simulink model "DC_motor_EX2_4"  (R2022a)
settings: Solver=FixedStepDiscrete  StartTime=0.0  StopTime=0.2  FixedStep=Ts  RelTol=1e-3  EnableMultiTasking=on
values from neighbouring files (symbols this model uses):
  Ad = dis_sys.A    [DC_motor.m]
  B_noise1 = [Bd Bw]    [DC_motor.m]
  Bd = dis_sys.B    [DC_motor.m]
  Cd = dis_sys.C    [DC_motor.m]
  D_noise1 = [Dd Dd Dd]    [DC_motor.m]
  N = 10    [DC_motor.m]
  P1 = zeros(size(S))    [DC_motor.m]
  Pr = P    [DC_motor.m]
  Q = 1000*eye(2)    [DC_motor.m]
  QMPC = Q    [DC_motor.m]
  R = R    (= 1)    [DC_motor.m]
  S = P    [DC_motor.m]
  sat_max = Vmax    (= 12)    [DC_motor.m]
  sat_min = Vmin    (= 0)    [DC_motor.m]
  Ts = 1e-3    (= 0.001)    [DC_motor.m]
  Vmax = 12    [DC_motor.m]
  Vmin = 0    [DC_motor.m]
  W = [1 ... (first row only)    [DC_motor.m]
  x0 = [I0 n0]'    [DC_motor.m]
  xmax = [Imax,nmax]'    [DC_motor.m]
  xmin = [Imin,nmin]'    [DC_motor.m]
  xref = [0 0]'    [DC_motor.m]
undefined symbols (not defined in the file or in its folder): MPC_Constrainte, mympc
settings Model: Creator=Mirko  LastModifiedBy=jj
settings SolverCC: AlgebraicLoopSolver=TrustRegion
settings DataIOCC: LimitDataPoints=on  SaveFormat=Array  SignalLoggingSaveFormat=ModelDataLogs  ReturnWorkspaceOutputs=off
settings OptimizationCC: ExpressionDepthLimit=2147483647  LifeSpan=inf
settings DebuggingCC: UnderspecifiedInitializationDetection=Classic  MergeDetectMultiDrivingBlocksExec=none  SolverPrmCheckMsg=warning  FcnCallInpInsideContextMsg=warning  UnconnectedInputMsg=warning  UnconnectedOutputMsg=warning  UnconnectedLineMsg=warning  StateNameClashWarn=warning  SFUnexpectedBacktrackingDiag=warning  SFNoUnconditionalDefaultTransitionDiag=warning  SFExecutionAtInitializationDiag=none  SFMachineParentedDataDiag=warning  ArithmeticOperatorsInVariantConditions=warning
settings HardwareCC: ProdBitPerPointer=32  ProdBitPerSizeT=32  ProdBitPerPtrDiffT=32  ProdLargestAtomicFloat=None  ProdIntDivRoundTo=Undefined  ProdEndianess=Unspecified  ProdWordSize=32  ProdHWDeviceType=32-bit Generic
settings ModelReferenceCC: PropagateSignalLabelsOutOfModel=off
settings SFSimCC: SimUseLocalCustomCode=off  CustomCodeUndefinedFunction=UseInterfaceOnly
settings RTWCC: RTWUseLocalCustomCode=off  DLArmComputeVersion=19.05
settings CodeAppCC: StateflowObjectComments=on
settings GRTTargetCC: TargetLangStandard=C89/C90 (ANSI)
settings ConfigComp: CovMetricSettings=dw  CovSaveCumulativeToWorkspaceVar=on  CovSaveSingleToWorkspaceVar=on  CovExternalEMLEnable=off  CovSFcnEnable=off

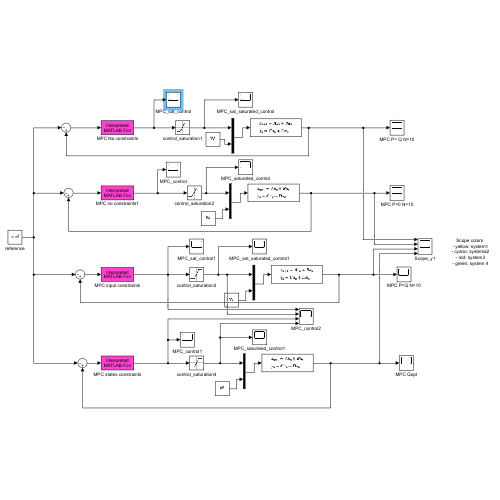
[thumbnail: Simulink's stored preview of the top-level diagram]
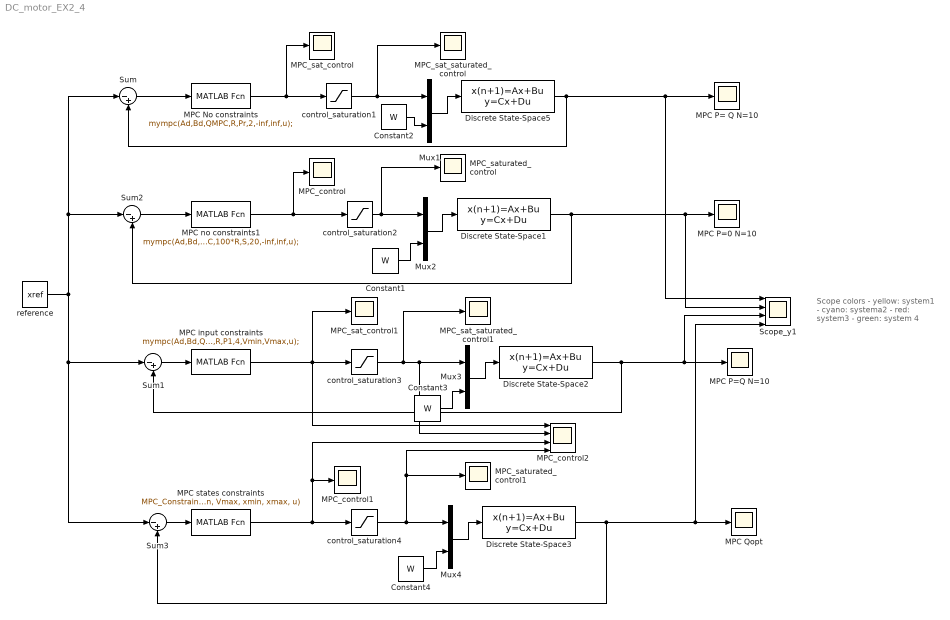
== system DC_motor_EX2_4 ==
  note: Scope colors
      | - yellow: system1
      | - cyano: systema2
      | - red: system3
      | - green: system 4
  Constant{1..4} (4 alike) : Constant  Value=W  SampleTime=Ts
  Discrete State-Space{1..3,5} (4 alike) : DiscreteStateSpace  A=Ad  B=B_noise1  C=Cd  D=D_noise1  InitialCondition=x0  SampleTime=Ts
  MPC No constraints : MATLABFcn  MATLABFcn=mympc(Ad,Bd,QMPC,R,Pr,2,-inf,inf,u);  OutputDimensions=1
  MPC P= Q N=10 : Scope
  MPC P=0 N=10 : Scope
  MPC P=Q N=10 : Scope
  MPC Qopt : Scope
  MPC input constraints : MATLABFcn  MATLABFcn=mympc(Ad,Bd,QMPC,R,P1,4,Vmin,Vmax,u);  OutputDimensions=1
  MPC no constraints1 : MATLABFcn  MATLABFcn=mympc(Ad,Bd,QMPC,100*R,S,20,-inf,inf,u);  OutputDimensions=1
  MPC states constraints : MATLABFcn  MATLABFcn=MPC_Constrainte( Ad,Bd, Q, R, Pr, N, Vmin, Vmax, xmin, xmax, u)  OutputDimensions=1
  MPC_control : Scope
  MPC_control1 : Scope
  MPC_control2 : Scope  NumInputPorts=4
  MPC_sat_control : Scope
  MPC_sat_control1 : Scope
  MPC_sat_saturated_control : Scope
  MPC_sat_saturated_control1 : Scope
  MPC_saturated_control : Scope
  MPC_saturated_control1 : Scope
  Mux{1..4} (4 alike) : Mux  Inputs=2
  Scope_y1 : Scope  NumInputPorts=4
  Sum{,1..3} (4 alike) : Sum  Inputs=|-+
  control_saturation1 : Saturate  UpperLimit=inf  LowerLimit=-inf
  control_saturation2 : Saturate  UpperLimit=inf  LowerLimit=-inf
  control_saturation3 : Saturate  UpperLimit=sat_max  LowerLimit=sat_min
  control_saturation4 : Saturate  UpperLimit=sat_max  LowerLimit=sat_min
  reference : Constant  Value=xref
  wires:
  Sum/1 -> MPC No constraints/1
  MPC No constraints/1 -> control_saturation1/1, MPC_sat_control/1
  Discrete State-Space5/1 -> MPC P= Q N=10/1, Scope_y1/1, Sum/2
  MPC no constraints1/1 -> control_saturation2/1, MPC_control/1
  Discrete State-Space1/1 -> Scope_y1/2, MPC P=0 N=10/1, Sum2/2
  Sum2/1 -> MPC no constraints1/1
  Sum3/1 -> MPC states constraints/1
  control_saturation4/1 -> Mux4/1, MPC_control2/4, MPC_saturated_control1/1
  Discrete State-Space3/1 -> MPC Qopt/1, Scope_y1/4, Sum3/2
  MPC states constraints/1 -> control_saturation4/1, MPC_control2/3, MPC_control1/1
  Discrete State-Space2/1 -> Sum1/2, Scope_y1/3, MPC P=Q N=10/1
  control_saturation3/1 -> Mux3/1, MPC_control2/2, MPC_sat_saturated_control1/1
  MPC input constraints/1 -> MPC_control2/1, control_saturation3/1, MPC_sat_control1/1
  Sum1/1 -> MPC input constraints/1
  reference/1 -> Sum1/1, Sum3/1, Sum/1, Sum2/1
  Mux1/1 -> Discrete State-Space5/1
  Constant2/1 -> Mux1/2
  control_saturation1/1 -> Mux1/1, MPC_sat_saturated_control/1
  Constant1/1 -> Mux2/2
  Mux2/1 -> Discrete State-Space1/1
  control_saturation2/1 -> Mux2/1, MPC_saturated_control/1
  Constant3/1 -> Mux3/2
  Mux3/1 -> Discrete State-Space2/1
  Constant4/1 -> Mux4/2
  Mux4/1 -> Discrete State-Space3/1
